simulink model "DLL_Demo"  (R2021a)
settings: Solver=VariableStepAuto  StartTime=0.0  StopTime=inf  RelTol=1e-3
settings Model: Creator=ccortez  LastModifiedBy=jdehg
settings SolverCC: AlgebraicLoopSolver=TrustRegion
settings DebuggingCC: SFMachineParentedDataDiag=warning

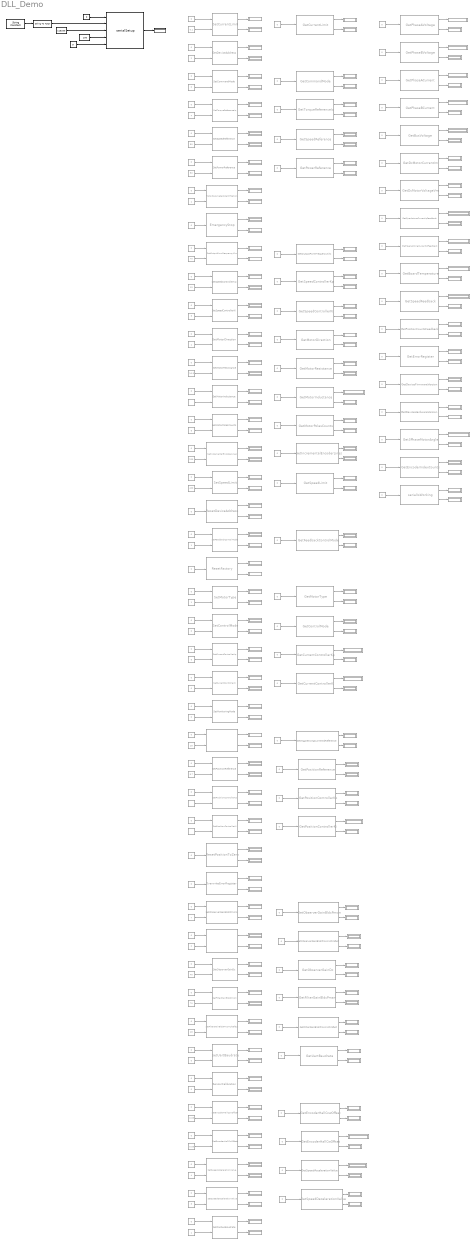
== system DLL_Demo ==
  note: Subsystem
  Constant1 : Constant  Value=115200  OutDataTypeStr=uint32
  Constant10 : Constant  Commented=on  Value=4  OutDataTypeStr=single
  Constant{2..3,6,8..9,11,15,17,19,21,23..24,26,28,30,32,34,36,38,40,42..43,45..48,50,52,54,56,58,60,62..64,66,68,70,72,74,76..78,80,82,84,86,88..136} (96 alike) : Constant  Commented=on  Value=0  OutDataTypeStr=uint8
  Constant12 : Constant  Value=100  OutDataTypeStr=double
  Constant13 : Constant  Value=5  OutDataTypeStr=int32
  Constant14 : Constant  Commented=on  Value=50  OutDataTypeStr=uint32
  Constant16 : Constant  Commented=on  Value=50  OutDataTypeStr=single
  Constant18 : Constant  Value=0  OutDataTypeStr=uint8
  Constant20 : Constant  Commented=on  OutDataTypeStr=boolean
  Constant22 : Constant  Commented=on  Value=70  OutDataTypeStr=uint32
  Constant25 : Constant  Commented=on  Value=13  OutDataTypeStr=single
  Constant27 : Constant  Commented=on  Value=9  OutDataTypeStr=single
  Constant29 : Constant  Commented=on  OutDataTypeStr=boolean
  Constant31 : Constant  Commented=on  Value=10.5  OutDataTypeStr=single
  Constant33 : Constant  Commented=on  Value=0.004  OutDataTypeStr=single
  Constant35 : Constant  Commented=on  Value=6  OutDataTypeStr=uint32
  Constant37 : Constant  Commented=on  Value=200  OutDataTypeStr=uint32
  Constant39 : Constant  Commented=on  Value=400  OutDataTypeStr=uint32
  Constant4 : Constant  Commented=on  Value=0.1  OutDataTypeStr=single
  Constant41 : Constant  Commented=on  OutDataTypeStr=uint8
  Constant44 : Constant  Commented=on  OutDataTypeStr=uint8
  Constant49 : Constant  Commented=on  Value=6  OutDataTypeStr=single
  Constant5 : Constant  Commented=on  Value=2  OutDataTypeStr=uint8
  Constant51 : Constant  Commented=on  Value=0  OutDataTypeStr=single
  Constant53 : Constant  Commented=on  Value=0  OutDataTypeStr=boolean
  Constant55 : Constant  Commented=on  Value=18  OutDataTypeStr=single
  Constant57 : Constant  Commented=on  Value=5.7  OutDataTypeStr=uint32
  Constant59 : Constant  Commented=on  Value=16.78  OutDataTypeStr=single
  Constant61 : Constant  Commented=on  Value=10.76  OutDataTypeStr=single
  Constant65 : Constant  Commented=on  Value=7  OutDataTypeStr=single
  Constant67 : Constant  Commented=on  Value=2  OutDataTypeStr=single
  Constant69 : Constant  Commented=on  Value=40  OutDataTypeStr=single
  Constant7 : Constant  Commented=on  Value=0  OutDataTypeStr=boolean
  Constant71 : Constant  Commented=on  Value=70  OutDataTypeStr=single
  Constant73 : Constant  Commented=on  Value=18  OutDataTypeStr=single
  Constant75 : Constant  Commented=on  Value=0  OutDataTypeStr=boolean
  Constant79 : Constant  Commented=on  Value=0.05  OutDataTypeStr=single
  Constant81 : Constant  Commented=on  Value=0.05  OutDataTypeStr=single
  Constant83 : Constant  Commented=on  Value=4  OutDataTypeStr=single
  Constant85 : Constant  Commented=on  Value=3  OutDataTypeStr=single
  Constant87 : Constant  Commented=on  OutDataTypeStr=uint8
  Display{1..4,6..189} (188 alike) : Display  Commented=on
      settings: Format=decimal (Stored Integer)
  Display5 : Display
      settings: Format=decimal (Stored Integer)
  S-Function Builder : S-Function  Priority=2  Commented=on  FunctionName=SetCurrentLimit  SFunctionModules=SetCurrentLimit_wrapper  SFunctionDeploymentMode=off  EnableBusSupport=off  mask(S-Function Builder){}
      mask help: Simulink:masks:SFunctionBuilder_MD
      mask init:
      | val = [[.9  0.75 0.75 1 1 .9 .9 1]',[1 1 0.75 0.75 .9 .9 1 .9]'];try , sys = get_param(gcb,'SfunBuilderFcnName');if isempty(sys), sys = get_param(gcb,'FunctionName'); end,catch, sys = get_param(gcb,'FunctionName'); end
      settings: CopyFcn=set_param(gcbh,'LinkStatus','none')  OpenFcn=sfunctionwizard(gcbh)
      mask Display: plot(val(:,1),val(:,2)),disp(sys),port_label('input',1,'Address'),port_label('input',2,'Value'),port_label('output',1,'Result'),port_label('output',2,'Error')
  S-Function Builder1 : S-Function  Priority=2  Commented=on  FunctionName=SetDeviceAddress  SFunctionModules=SetDeviceAddress_wrapper  SFunctionDeploymentMode=off  EnableBusSupport=off  mask(S-Function Builder){}
      mask help: Simulink:masks:SFunctionBuilder_MD
      mask init: same as DLL_Demo/S-Function Builder
      settings: CopyFcn=set_param(gcbh,'LinkStatus','none')  OpenFcn=sfunctionwizard(gcbh)
      mask Display: plot(val(:,1),val(:,2)),disp(sys),port_label('input',1,'Address'),port_label('input',2,'Value'),port_label('output',1,'Result'),port_label('output',2,'Error')
  S-Function Builder10 : S-Function  Priority=2  Commented=on  FunctionName=MotorParametersIdentification  SFunctionModules=MotorParametersIdentification_wrapper  SFunctionDeploymentMode=off  EnableBusSupport=off  mask(S-Function Builder){}
      mask help: Simulink:masks:SFunctionBuilder_MD
      mask init: same as DLL_Demo/S-Function Builder
      settings: CopyFcn=set_param(gcbh,'LinkStatus','none')  OpenFcn=sfunctionwizard(gcbh)
      mask Display: plot(val(:,1),val(:,2)),disp(sys),port_label('input',1,'Address'),port_label('input',2,'Value'),port_label('output',1,'Result'),port_label('output',2,'Error')
  S-Function Builder11 : S-Function  Priority=2  Commented=on  FunctionName=EmergencyStop  SFunctionModules=EmergencyStop_wrapper  SFunctionDeploymentMode=off  EnableBusSupport=off  mask(S-Function Builder){}
      mask help: Simulink:masks:SFunctionBuilder_MD
      mask init: same as DLL_Demo/S-Function Builder
      settings: CopyFcn=set_param(gcbh,'LinkStatus','none')  OpenFcn=sfunctionwizard(gcbh)
      mask Display:
      | plot(val(:,1),val(:,2))
      | disp(sys)
      | port_label('input',1,'Address')
      | port_label('output',1,'Result')
      | port_label('output',2,'Error')
  S-Function Builder12 : S-Function  Priority=2  Commented=on  FunctionName=SetOutputPwmFrequencyKhz  SFunctionModules=SetOutputPwmFrequencyKhz_wrapper  SFunctionDeploymentMode=off  EnableBusSupport=off  mask(S-Function Builder){}
      mask help: Simulink:masks:SFunctionBuilder_MD
      mask init: same as DLL_Demo/S-Function Builder
      settings: CopyFcn=set_param(gcbh,'LinkStatus','none')  OpenFcn=sfunctionwizard(gcbh)
      mask Display:
      | plot(val(:,1),val(:,2))
      | disp(sys)
      | port_label('input',1,'Address')
      | port_label('input',2,'Value')
      | port_label('output',1,'Result')
      | port_label('output',2,'Error')
  S-Function Builder13 : S-Function  Priority=2  Commented=on  FunctionName=SetSpeedControllerKp  SFunctionModules=SetSpeedControllerKp_wrapper  SFunctionDeploymentMode=off  EnableBusSupport=off  mask(S-Function Builder){}
      mask help: Simulink:masks:SFunctionBuilder_MD
      mask init: same as DLL_Demo/S-Function Builder
      settings: CopyFcn=set_param(gcbh,'LinkStatus','none')  OpenFcn=sfunctionwizard(gcbh)
      mask Display: plot(val(:,1),val(:,2)),disp(sys),port_label('input',1,'Address'),port_label('input',2,'Value'),port_label('output',1,'Result'),port_label('output',2,'Error')
  S-Function Builder14 : S-Function  Priority=2  Commented=on  FunctionName=SetSpeedControllerKi  SFunctionModules=SetSpeedControllerKi_wrapper  SFunctionDeploymentMode=off  EnableBusSupport=off  mask(S-Function Builder){}
      mask help: Simulink:masks:SFunctionBuilder_MD
      mask init: same as DLL_Demo/S-Function Builder
      settings: CopyFcn=set_param(gcbh,'LinkStatus','none')  OpenFcn=sfunctionwizard(gcbh)
      mask Display: plot(val(:,1),val(:,2)),disp(sys),port_label('input',1,'Address'),port_label('input',2,'Value'),port_label('output',1,'Result'),port_label('output',2,'Error')
  S-Function Builder15 : S-Function  Priority=2  Commented=on  FunctionName=SetMotorDirection  SFunctionModules=SetMotorDirection_wrapper  SFunctionDeploymentMode=off  EnableBusSupport=off  mask(S-Function Builder){}
      mask help: Simulink:masks:SFunctionBuilder_MD
      mask init: same as DLL_Demo/S-Function Builder
      settings: CopyFcn=set_param(gcbh,'LinkStatus','none')  OpenFcn=sfunctionwizard(gcbh)
      mask Display: plot(val(:,1),val(:,2)),disp(sys),port_label('input',1,'Address'),port_label('input',2,'Value'),port_label('output',1,'Result'),port_label('output',2,'Error')
  S-Function Builder16 : S-Function  Priority=2  Commented=on  FunctionName=SetMotorResistance  SFunctionModules=SetMotorResistance_wrapper  SFunctionDeploymentMode=off  EnableBusSupport=off  mask(S-Function Builder){}
      mask help: Simulink:masks:SFunctionBuilder_MD
      mask init: same as DLL_Demo/S-Function Builder
      settings: CopyFcn=set_param(gcbh,'LinkStatus','none')  OpenFcn=sfunctionwizard(gcbh)
      mask Display: plot(val(:,1),val(:,2)),disp(sys),port_label('input',1,'Address'),port_label('input',2,'Value'),port_label('output',1,'Result'),port_label('output',2,'Error')
  S-Function Builder17 : S-Function  Priority=2  Commented=on  FunctionName=SetMotorInductance  SFunctionModules=SetMotorInductance_wrapper  SFunctionDeploymentMode=off  EnableBusSupport=off  mask(S-Function Builder){}
      mask help: Simulink:masks:SFunctionBuilder_MD
      mask init: same as DLL_Demo/S-Function Builder
      settings: CopyFcn=set_param(gcbh,'LinkStatus','none')  OpenFcn=sfunctionwizard(gcbh)
      mask Display: plot(val(:,1),val(:,2)),disp(sys),port_label('input',1,'Address'),port_label('input',2,'Value'),port_label('output',1,'Result'),port_label('output',2,'Error')
  S-Function Builder18 : S-Function  Priority=2  Commented=on  FunctionName=SetMotorPolesCounts  SFunctionModules=SetMotorPolesCounts_wrapper  SFunctionDeploymentMode=off  EnableBusSupport=off  mask(S-Function Builder){}
      mask help: Simulink:masks:SFunctionBuilder_MD
      mask init: same as DLL_Demo/S-Function Builder
      settings: CopyFcn=set_param(gcbh,'LinkStatus','none')  OpenFcn=sfunctionwizard(gcbh)
      mask Display:
      | plot(val(:,1),val(:,2))
      | disp(sys)
      | port_label('input',1,'Address')
      | port_label('input',2,'Value')
      | port_label('output',1,'Result')
      | port_label('output',2,'Error')
  S-Function Builder19 : S-Function  Priority=2  Commented=on  FunctionName=SetIncrementalEncoderLines  SFunctionModules=SetIncrementalEncoderLines_wrapper  SFunctionDeploymentMode=off  EnableBusSupport=off  mask(S-Function Builder){}
      mask help: Simulink:masks:SFunctionBuilder_MD
      mask init: same as DLL_Demo/S-Function Builder
      settings: CopyFcn=set_param(gcbh,'LinkStatus','none')  OpenFcn=sfunctionwizard(gcbh)
      mask Display:
      | plot(val(:,1),val(:,2))
      | disp(sys)
      | port_label('input',1,'Address')
      | port_label('input',2,'Value')
      | port_label('output',1,'Result')
      | port_label('output',2,'Error')
  S-Function Builder2 : S-Function  Priority=2  Commented=on  FunctionName=SetCommandMode  SFunctionModules=SetCommandMode_wrapper  SFunctionDeploymentMode=off  EnableBusSupport=off  mask(S-Function Builder){}
      mask help: Simulink:masks:SFunctionBuilder_MD
      mask init: same as DLL_Demo/S-Function Builder
      settings: CopyFcn=set_param(gcbh,'LinkStatus','none')  OpenFcn=sfunctionwizard(gcbh)
      mask Display: plot(val(:,1),val(:,2)),disp(sys),port_label('input',1,'Address'),port_label('input',2,'Value'),port_label('output',1,'Result'),port_label('output',2,'Error')
  S-Function Builder20 : S-Function  Priority=2  Commented=on  FunctionName=SetSpeedLimit  SFunctionModules=SetSpeedLimit_wrapper  SFunctionDeploymentMode=off  EnableBusSupport=off  mask(S-Function Builder){}
      mask help: Simulink:masks:SFunctionBuilder_MD
      mask init: same as DLL_Demo/S-Function Builder
      settings: CopyFcn=set_param(gcbh,'LinkStatus','none')  OpenFcn=sfunctionwizard(gcbh)
      mask Display:
      | plot(val(:,1),val(:,2))
      | disp(sys)
      | port_label('input',1,'Address')
      | port_label('input',2,'Value')
      | port_label('output',1,'Result')
      | port_label('output',2,'Error')
  S-Function Builder21 : S-Function  Priority=2  Commented=on  FunctionName=SetFeedbackControlMode  SFunctionModules=SetFeedbackControlMode_wrapper  SFunctionDeploymentMode=off  EnableBusSupport=off  mask(S-Function Builder){}
      mask help: Simulink:masks:SFunctionBuilder_MD
      mask init: same as DLL_Demo/S-Function Builder
      settings: CopyFcn=set_param(gcbh,'LinkStatus','none')  OpenFcn=sfunctionwizard(gcbh)
      mask Display: plot(val(:,1),val(:,2)),disp(sys),port_label('input',1,'Address'),port_label('input',2,'Value'),port_label('output',1,'Result'),port_label('output',2,'Error')
  S-Function Builder22 : S-Function  Priority=2  Commented=on  FunctionName=ResetDeviceAddress  SFunctionModules=ResetDeviceAddress_wrapper  SFunctionDeploymentMode=off  EnableBusSupport=off  mask(S-Function Builder){}
      mask help: Simulink:masks:SFunctionBuilder_MD
      mask init: same as DLL_Demo/S-Function Builder
      settings: CopyFcn=set_param(gcbh,'LinkStatus','none')  OpenFcn=sfunctionwizard(gcbh)
      mask Display:
      | plot(val(:,1),val(:,2))
      | disp(sys)
      | port_label('input',1,'Address')
      | port_label('output',1,'Result')
      | port_label('output',2,'Error')
  S-Function Builder23 : S-Function  Priority=2  Commented=on  FunctionName=SetMotorType  SFunctionModules=SetMotorType_wrapper  SFunctionDeploymentMode=off  EnableBusSupport=off  mask(S-Function Builder){}
      mask help: Simulink:masks:SFunctionBuilder_MD
      mask init: same as DLL_Demo/S-Function Builder
      settings: CopyFcn=set_param(gcbh,'LinkStatus','none')  OpenFcn=sfunctionwizard(gcbh)
      mask Display: plot(val(:,1),val(:,2)),disp(sys),port_label('input',1,'Address'),port_label('input',2,'Value'),port_label('output',1,'Result'),port_label('output',2,'Error')
  S-Function Builder24 : S-Function  Priority=2  Commented=on  FunctionName=ResetFactory  SFunctionModules=ResetFactory_wrapper  SFunctionDeploymentMode=off  EnableBusSupport=off  mask(S-Function Builder){}
      mask help: Simulink:masks:SFunctionBuilder_MD
      mask init: same as DLL_Demo/S-Function Builder
      settings: CopyFcn=set_param(gcbh,'LinkStatus','none')  OpenFcn=sfunctionwizard(gcbh)
      mask Display:
      | plot(val(:,1),val(:,2))
      | disp(sys)
      | port_label('input',1,'Address')
      | port_label('output',1,'Result')
      | port_label('output',2,'Error')
  S-Function Builder25 : S-Function  Priority=2  Commented=on  FunctionName=SetControlMode  SFunctionModules=SetControlMode_wrapper  SFunctionDeploymentMode=off  EnableBusSupport=off  mask(S-Function Builder){}
      mask help: Simulink:masks:SFunctionBuilder_MD
      mask init: same as DLL_Demo/S-Function Builder
      settings: CopyFcn=set_param(gcbh,'LinkStatus','none')  OpenFcn=sfunctionwizard(gcbh)
      mask Display: plot(val(:,1),val(:,2)),disp(sys),port_label('input',1,'Address'),port_label('input',2,'Value'),port_label('output',1,'Result'),port_label('output',2,'Error')
  S-Function Builder26 : S-Function  Priority=2  Commented=on  FunctionName=SetCurrentControllerKp  SFunctionModules=SetCurrentControllerKp_wrapper  SFunctionDeploymentMode=off  EnableBusSupport=off  mask(S-Function Builder){}
      mask help: Simulink:masks:SFunctionBuilder_MD
      mask init: same as DLL_Demo/S-Function Builder
      settings: CopyFcn=set_param(gcbh,'LinkStatus','none')  OpenFcn=sfunctionwizard(gcbh)
      mask Display: plot(val(:,1),val(:,2)),disp(sys),port_label('input',1,'Address'),port_label('input',2,'Value'),port_label('output',1,'Result'),port_label('output',2,'Error')
  S-Function Builder27 : S-Function  Priority=2  Commented=on  FunctionName=SetCurrentControllerKi  SFunctionModules=SetCurrentControllerKi_wrapper  SFunctionDeploymentMode=off  EnableBusSupport=off  mask(S-Function Builder){}
      mask help: Simulink:masks:SFunctionBuilder_MD
      mask init: same as DLL_Demo/S-Function Builder
      settings: CopyFcn=set_param(gcbh,'LinkStatus','none')  OpenFcn=sfunctionwizard(gcbh)
      mask Display: plot(val(:,1),val(:,2)),disp(sys),port_label('input',1,'Address'),port_label('input',2,'Value'),port_label('output',1,'Result'),port_label('output',2,'Error')
  S-Function Builder28 : S-Function  Priority=2  Commented=on  FunctionName=SetMonitoringMode  SFunctionModules=SetMonitoringMode_wrapper  SFunctionDeploymentMode=off  EnableBusSupport=off  mask(S-Function Builder){}
      mask help: Simulink:masks:SFunctionBuilder_MD
      mask init: same as DLL_Demo/S-Function Builder
      settings: CopyFcn=set_param(gcbh,'LinkStatus','none')  OpenFcn=sfunctionwizard(gcbh)
      mask Display: plot(val(:,1),val(:,2)),disp(sys),port_label('input',1,'Address'),port_label('input',2,'Value'),port_label('output',1,'Result'),port_label('output',2,'Error')
  S-Function Builder29 : S-Function  Priority=2  Commented=on  FunctionName=SetMagnetizingCurrentIdReference  SFunctionModules=SetMagnetizingCurrentIdReference_wrapper  SFunctionDeploymentMode=off  EnableBusSupport=off  mask(S-Function Builder){}
      mask help: Simulink:masks:SFunctionBuilder_MD
      mask init: same as DLL_Demo/S-Function Builder
      settings: CopyFcn=set_param(gcbh,'LinkStatus','none')  OpenFcn=sfunctionwizard(gcbh)
      mask Display: plot(val(:,1),val(:,2)),disp(sys),port_label('input',1,'Address'),port_label('input',2,'Value'),port_label('output',1,'Result'),port_label('output',2,'Error')
  S-Function Builder3 : S-Function  Priority=3  Commented=on  FunctionName=GetCommandMode  SFunctionModules=GetCommandMode_wrapper  SFunctionDeploymentMode=off  EnableBusSupport=off  mask(S-Function Builder){}
      mask help: Simulink:masks:SFunctionBuilder_MD
      mask init: same as DLL_Demo/S-Function Builder
      settings: CopyFcn=set_param(gcbh,'LinkStatus','none')  OpenFcn=sfunctionwizard(gcbh)
      mask Display: plot(val(:,1),val(:,2)),disp(sys),port_label('input',1,'Address'),port_label('output',1,'Result'),port_label('output',2,'Error')
  S-Function Builder30 : S-Function  Priority=2  Commented=on  FunctionName=SetPositionReference  SFunctionModules=SetPositionReference_wrapper  SFunctionDeploymentMode=off  EnableBusSupport=off  mask(S-Function Builder){}
      mask help: Simulink:masks:SFunctionBuilder_MD
      mask init: same as DLL_Demo/S-Function Builder
      settings: CopyFcn=set_param(gcbh,'LinkStatus','none')  OpenFcn=sfunctionwizard(gcbh)
      mask Display:
      | plot(val(:,1),val(:,2))
      | disp(sys)
      | port_label('input',1,'Address')
      | port_label('input',2,'Value')
      | port_label('output',1,'Result')
      | port_label('output',2,'Error')
  S-Function Builder31 : S-Function  Priority=2  Commented=on  FunctionName=SetPositionControllerKp  SFunctionModules=SetPositionControllerKp_wrapper  SFunctionDeploymentMode=off  EnableBusSupport=off  mask(S-Function Builder){}
      mask help: Simulink:masks:SFunctionBuilder_MD
      mask init: same as DLL_Demo/S-Function Builder
      settings: CopyFcn=set_param(gcbh,'LinkStatus','none')  OpenFcn=sfunctionwizard(gcbh)
      mask Display: plot(val(:,1),val(:,2)),disp(sys),port_label('input',1,'Address'),port_label('input',2,'Value'),port_label('output',1,'Result'),port_label('output',2,'Error')
  S-Function Builder32 : S-Function  Priority=2  Commented=on  FunctionName=SetPositionControllerKi  SFunctionModules=SetPositionControllerKi_wrapper  SFunctionDeploymentMode=off  EnableBusSupport=off  mask(S-Function Builder){}
      mask help: Simulink:masks:SFunctionBuilder_MD
      mask init: same as DLL_Demo/S-Function Builder
      settings: CopyFcn=set_param(gcbh,'LinkStatus','none')  OpenFcn=sfunctionwizard(gcbh)
      mask Display: plot(val(:,1),val(:,2)),disp(sys),port_label('input',1,'Address'),port_label('input',2,'Value'),port_label('output',1,'Result'),port_label('output',2,'Error')
  S-Function Builder33 : S-Function  Priority=2  Commented=on  FunctionName=ResetPositionToZero  SFunctionModules=ResetPositionToZero_wrapper  SFunctionDeploymentMode=off  EnableBusSupport=off  mask(S-Function Builder){}
      mask help: Simulink:masks:SFunctionBuilder_MD
      mask init: same as DLL_Demo/S-Function Builder
      settings: CopyFcn=set_param(gcbh,'LinkStatus','none')  OpenFcn=sfunctionwizard(gcbh)
      mask Display:
      | plot(val(:,1),val(:,2))
      | disp(sys)
      | port_label('input',1,'Address')
      | port_label('output',1,'Result')
      | port_label('output',2,'Error')
  S-Function Builder34 : S-Function  Priority=2  Commented=on  FunctionName=OverwriteErrorRegister  SFunctionModules=OverwriteErrorRegister_wrapper  SFunctionDeploymentMode=off  EnableBusSupport=off  mask(S-Function Builder){}
      mask help: Simulink:masks:SFunctionBuilder_MD
      mask init: same as DLL_Demo/S-Function Builder
      settings: CopyFcn=set_param(gcbh,'LinkStatus','none')  OpenFcn=sfunctionwizard(gcbh)
      mask Display:
      | plot(val(:,1),val(:,2))
      | disp(sys)
      | port_label('input',1,'Address')
      | port_label('output',1,'Result')
      | port_label('output',2,'Error')
  S-Function Builder35 : S-Function  Priority=2  Commented=on  FunctionName=SetObserverGainBldcPmsm  SFunctionModules=SetObserverGainBldcPmsm_wrapper  SFunctionDeploymentMode=off  EnableBusSupport=off  mask(S-Function Builder){}
      mask help: Simulink:masks:SFunctionBuilder_MD
      mask init: same as DLL_Demo/S-Function Builder
      settings: CopyFcn=set_param(gcbh,'LinkStatus','none')  OpenFcn=sfunctionwizard(gcbh)
      mask Display: plot(val(:,1),val(:,2)),disp(sys),port_label('input',1,'Address'),port_label('input',2,'Value'),port_label('output',1,'Result'),port_label('output',2,'Error')
  S-Function Builder36 : S-Function  Priority=2  Commented=on  FunctionName=SetObserverGainBldcPmsmUltrafast  SFunctionModules=SetObserverGainBldcPmsmUltrafast_wrapper  SFunctionDeploymentMode=off  EnableBusSupport=off  mask(S-Function Builder){}
      mask help: Simulink:masks:SFunctionBuilder_MD
      mask init: same as DLL_Demo/S-Function Builder
      settings: CopyFcn=set_param(gcbh,'LinkStatus','none')  OpenFcn=sfunctionwizard(gcbh)
      mask Display: plot(val(:,1),val(:,2)),disp(sys),port_label('input',1,'Address'),port_label('input',2,'Value'),port_label('output',1,'Result'),port_label('output',2,'Error')
  S-Function Builder37 : S-Function  Priority=2  Commented=on  FunctionName=SetObserverGainDc  SFunctionModules=SetObserverGainDc_wrapper  SFunctionDeploymentMode=off  EnableBusSupport=off  mask(S-Function Builder){}
      mask help: Simulink:masks:SFunctionBuilder_MD
      mask init: same as DLL_Demo/S-Function Builder
      settings: CopyFcn=set_param(gcbh,'LinkStatus','none')  OpenFcn=sfunctionwizard(gcbh)
      mask Display: plot(val(:,1),val(:,2)),disp(sys),port_label('input',1,'Address'),port_label('input',2,'Value'),port_label('output',1,'Result'),port_label('output',2,'Error')
  S-Function Builder38 : S-Function  Priority=2  Commented=on  FunctionName=SetFilterGainBldcPmsm  SFunctionModules=SetFilterGainBldcPmsm_wrapper  SFunctionDeploymentMode=off  EnableBusSupport=off  mask(S-Function Builder){}
      mask help: Simulink:masks:SFunctionBuilder_MD
      mask init: same as DLL_Demo/S-Function Builder
      settings: CopyFcn=set_param(gcbh,'LinkStatus','none')  OpenFcn=sfunctionwizard(gcbh)
      mask Display: plot(val(:,1),val(:,2)),disp(sys),port_label('input',1,'Address'),port_label('input',2,'Value'),port_label('output',1,'Result'),port_label('output',2,'Error')
  S-Function Builder39 : S-Function  Priority=2  Commented=on  FunctionName=SetFilterGainBldcPmsmUltrafast  SFunctionModules=SetFilterGainBldcPmsmUltrafast_wrapper  SFunctionDeploymentMode=off  EnableBusSupport=off  mask(S-Function Builder){}
      mask help: Simulink:masks:SFunctionBuilder_MD
      mask init: same as DLL_Demo/S-Function Builder
      settings: CopyFcn=set_param(gcbh,'LinkStatus','none')  OpenFcn=sfunctionwizard(gcbh)
      mask Display: plot(val(:,1),val(:,2)),disp(sys),port_label('input',1,'Address'),port_label('input',2,'Value'),port_label('output',1,'Result'),port_label('output',2,'Error')
  S-Function Builder4 : S-Function  Priority=2  Commented=on  FunctionName=SetTorqueReferenceIq  SFunctionModules=SetTorqueReferenceIq_wrapper  SFunctionDeploymentMode=off  EnableBusSupport=off  mask(S-Function Builder){}
      mask help: Simulink:masks:SFunctionBuilder_MD
      mask init: same as DLL_Demo/S-Function Builder
      settings: CopyFcn=set_param(gcbh,'LinkStatus','none')  OpenFcn=sfunctionwizard(gcbh)
      mask Display: plot(val(:,1),val(:,2)),disp(sys),port_label('input',1,'Address'),port_label('input',2,'Value'),port_label('output',1,'Result'),port_label('output',2,'Error')
  S-Function Builder40 : S-Function  Priority=2  Commented=on  FunctionName=SetUartBaudrate  SFunctionModules=SetUartBaudrate_wrapper  SFunctionDeploymentMode=off  EnableBusSupport=off  mask(S-Function Builder){}
      mask help: Simulink:masks:SFunctionBuilder_MD
      mask init: same as DLL_Demo/S-Function Builder
      settings: CopyFcn=set_param(gcbh,'LinkStatus','none')  OpenFcn=sfunctionwizard(gcbh)
      mask Display: plot(val(:,1),val(:,2)),disp(sys),port_label('input',1,'Address'),port_label('input',2,'Value'),port_label('output',1,'Result'),port_label('output',2,'Error')
  S-Function Builder41 : S-Function  Priority=2  Commented=on  FunctionName=SensorCalibration  SFunctionModules=SensorCalibration_wrapper  SFunctionDeploymentMode=off  EnableBusSupport=off  mask(S-Function Builder){}
      mask help: Simulink:masks:SFunctionBuilder_MD
      mask init: same as DLL_Demo/S-Function Builder
      settings: CopyFcn=set_param(gcbh,'LinkStatus','none')  OpenFcn=sfunctionwizard(gcbh)
      mask Display: plot(val(:,1),val(:,2)),disp(sys),port_label('input',1,'Address'),port_label('input',2,'Value'),port_label('output',1,'Result'),port_label('output',2,'Error')
  S-Function Builder42 : S-Function  Priority=2  Commented=on  FunctionName=SetEncoderHallCcwOffset  SFunctionModules=SetEncoderHallCcwOffset_wrapper  SFunctionDeploymentMode=off  EnableBusSupport=off  mask(S-Function Builder){}
      mask help: Simulink:masks:SFunctionBuilder_MD
      mask init: same as DLL_Demo/S-Function Builder
      settings: CopyFcn=set_param(gcbh,'LinkStatus','none')  OpenFcn=sfunctionwizard(gcbh)
      mask Display: plot(val(:,1),val(:,2)),disp(sys),port_label('input',1,'Address'),port_label('input',2,'Value'),port_label('output',1,'Result'),port_label('output',2,'Error')
  S-Function Builder43 : S-Function  Priority=2  Commented=on  FunctionName=SetEncoderHallCwOffset  SFunctionModules=SetEncoderHallCwOffset_wrapper  SFunctionDeploymentMode=off  EnableBusSupport=off  mask(S-Function Builder){}
      mask help: Simulink:masks:SFunctionBuilder_MD
      mask init: same as DLL_Demo/S-Function Builder
      settings: CopyFcn=set_param(gcbh,'LinkStatus','none')  OpenFcn=sfunctionwizard(gcbh)
      mask Display: plot(val(:,1),val(:,2)),disp(sys),port_label('input',1,'Address'),port_label('input',2,'Value'),port_label('output',1,'Result'),port_label('output',2,'Error')
  S-Function Builder44 : S-Function  Priority=2  Commented=on  FunctionName=SetSpeedAccelerationValue  SFunctionModules=SetSpeedAccelerationValue_wrapper  SFunctionDeploymentMode=off  EnableBusSupport=off  mask(S-Function Builder){}
      mask help: Simulink:masks:SFunctionBuilder_MD
      mask init: same as DLL_Demo/S-Function Builder
      settings: CopyFcn=set_param(gcbh,'LinkStatus','none')  OpenFcn=sfunctionwizard(gcbh)
      mask Display: plot(val(:,1),val(:,2)),disp(sys),port_label('input',1,'Address'),port_label('input',2,'Value'),port_label('output',1,'Result'),port_label('output',2,'Error')
  S-Function Builder45 : S-Function  Priority=2  Commented=on  FunctionName=SetSpeedDecelerationValue  SFunctionModules=SetSpeedDecelerationValue_wrapper  SFunctionDeploymentMode=off  EnableBusSupport=off  mask(S-Function Builder){}
      mask help: Simulink:masks:SFunctionBuilder_MD
      mask init: same as DLL_Demo/S-Function Builder
      settings: CopyFcn=set_param(gcbh,'LinkStatus','none')  OpenFcn=sfunctionwizard(gcbh)
      mask Display: plot(val(:,1),val(:,2)),disp(sys),port_label('input',1,'Address'),port_label('input',2,'Value'),port_label('output',1,'Result'),port_label('output',2,'Error')
  S-Function Builder46 : S-Function  Priority=2  Commented=on  FunctionName=SetCanbusBoudrate  SFunctionModules=SetCanbusBoudrate_wrapper  SFunctionDeploymentMode=off  EnableBusSupport=off  mask(S-Function Builder){}
      mask help: Simulink:masks:SFunctionBuilder_MD
      mask init: same as DLL_Demo/S-Function Builder
      settings: CopyFcn=set_param(gcbh,'LinkStatus','none')  OpenFcn=sfunctionwizard(gcbh)
      mask Display: plot(val(:,1),val(:,2)),disp(sys),port_label('input',1,'Address'),port_label('input',2,'Value'),port_label('output',1,'Result'),port_label('output',2,'Error')
  S-Function Builder47 : S-Function  Priority=3  Commented=on  FunctionName=GetPhaseAVoltage  SFunctionModules=GetPhaseAVoltage_wrapper  SFunctionDeploymentMode=off  EnableBusSupport=off  mask(S-Function Builder){}
      mask help: Simulink:masks:SFunctionBuilder_MD
      mask init: same as DLL_Demo/S-Function Builder
      settings: CopyFcn=set_param(gcbh,'LinkStatus','none')  OpenFcn=sfunctionwizard(gcbh)
      mask Display:
      | plot(val(:,1),val(:,2))
      | disp(sys)
      | port_label('input',1,'Address')
      | port_label('output',1,'Result')
      | port_label('output',2,'Error')
  S-Function Builder48 : S-Function  Priority=3  Commented=on  FunctionName=GetPhaseBVoltage  SFunctionModules=GetPhaseBVoltage_wrapper  SFunctionDeploymentMode=off  EnableBusSupport=off  mask(S-Function Builder){}
      mask help: Simulink:masks:SFunctionBuilder_MD
      mask init: same as DLL_Demo/S-Function Builder
      settings: CopyFcn=set_param(gcbh,'LinkStatus','none')  OpenFcn=sfunctionwizard(gcbh)
      mask Display:
      | plot(val(:,1),val(:,2))
      | disp(sys)
      | port_label('input',1,'Address')
      | port_label('output',1,'Result')
      | port_label('output',2,'Error')
  S-Function Builder49 : S-Function  Priority=3  Commented=on  FunctionName=GetPhaseACurrent  SFunctionModules=GetPhaseACurrent_wrapper  SFunctionDeploymentMode=off  EnableBusSupport=off  mask(S-Function Builder){}
      mask help: Simulink:masks:SFunctionBuilder_MD
      mask init: same as DLL_Demo/S-Function Builder
      settings: CopyFcn=set_param(gcbh,'LinkStatus','none')  OpenFcn=sfunctionwizard(gcbh)
      mask Display:
      | plot(val(:,1),val(:,2))
      | disp(sys)
      | port_label('input',1,'Address')
      | port_label('output',1,'Result')
      | port_label('output',2,'Error')
  S-Function Builder5 : S-Function  Priority=1  FunctionName=serialSetup  SFunctionModules=serialSetup_wrapper  SFunctionDeploymentMode=off  EnableBusSupport=off  mask(S-Function Builder){}
      mask help: Simulink:masks:SFunctionBuilder_MD
      mask init: same as DLL_Demo/S-Function Builder
      settings: CopyFcn=set_param(gcbh,'LinkStatus','none')  OpenFcn=sfunctionwizard(gcbh)
      mask Display: plot(val(:,1),val(:,2)),disp(sys),port_label('input',1,'Address'),port_label('input',2,'COM_Port'),port_label('input',3,'Baud_Rate'),port_label('input',4,'Timeout'),port_label('input',5,'Trials_on_Failure'),port_label('output',1,'Result')
  S-Function Builder50 : S-Function  Priority=3  Commented=on  FunctionName=GetPhaseBCurrent  SFunctionModules=GetPhaseBCurrent_wrapper  SFunctionDeploymentMode=off  EnableBusSupport=off  mask(S-Function Builder){}
      mask help: Simulink:masks:SFunctionBuilder_MD
      mask init: same as DLL_Demo/S-Function Builder
      settings: CopyFcn=set_param(gcbh,'LinkStatus','none')  OpenFcn=sfunctionwizard(gcbh)
      mask Display:
      | plot(val(:,1),val(:,2))
      | disp(sys)
      | port_label('input',1,'Address')
      | port_label('output',1,'Result')
      | port_label('output',2,'Error')
  S-Function Builder51 : S-Function  Priority=3  Commented=on  FunctionName=GetBusVoltage  SFunctionModules=GetBusVoltage_wrapper  SFunctionDeploymentMode=off  EnableBusSupport=off  mask(S-Function Builder){}
      mask help: Simulink:masks:SFunctionBuilder_MD
      mask init: same as DLL_Demo/S-Function Builder
      settings: CopyFcn=set_param(gcbh,'LinkStatus','none')  OpenFcn=sfunctionwizard(gcbh)
      mask Display:
      | plot(val(:,1),val(:,2))
      | disp(sys)
      | port_label('input',1,'Address')
      | port_label('output',1,'Result')
      | port_label('output',2,'Error')
  S-Function Builder52 : S-Function  Priority=3  Commented=on  FunctionName=GetDcMotorCurrentIm  SFunctionModules=GetDcMotorCurrentIm_wrapper  SFunctionDeploymentMode=off  EnableBusSupport=off  mask(S-Function Builder){}
      mask help: Simulink:masks:SFunctionBuilder_MD
      mask init: same as DLL_Demo/S-Function Builder
      settings: CopyFcn=set_param(gcbh,'LinkStatus','none')  OpenFcn=sfunctionwizard(gcbh)
      mask Display:
      | plot(val(:,1),val(:,2))
      | disp(sys)
      | port_label('input',1,'Address')
      | port_label('output',1,'Result')
      | port_label('output',2,'Error')
  S-Function Builder53 : S-Function  Priority=3  Commented=on  FunctionName=GetDcMotorVoltageVm  SFunctionModules=GetDcMotorVoltageVm_wrapper  SFunctionDeploymentMode=off  EnableBusSupport=off  mask(S-Function Builder){}
      mask help: Simulink:masks:SFunctionBuilder_MD
      mask init: same as DLL_Demo/S-Function Builder
      settings: CopyFcn=set_param(gcbh,'LinkStatus','none')  OpenFcn=sfunctionwizard(gcbh)
      mask Display:
      | plot(val(:,1),val(:,2))
      | disp(sys)
      | port_label('input',1,'Address')
      | port_label('output',1,'Result')
      | port_label('output',2,'Error')
  S-Function Builder54 : S-Function  Priority=3  Commented=on  FunctionName=GetSpeedControllerKp  SFunctionModules=GetSpeedControllerKp_wrapper  SFunctionDeploymentMode=off  EnableBusSupport=off  mask(S-Function Builder){}
      mask help: Simulink:masks:SFunctionBuilder_MD
      mask init: same as DLL_Demo/S-Function Builder
      settings: CopyFcn=set_param(gcbh,'LinkStatus','none')  OpenFcn=sfunctionwizard(gcbh)
      mask Display:
      | plot(val(:,1),val(:,2))
      | disp(sys)
      | port_label('input',1,'Address')
      | port_label('output',1,'Result')
      | port_label('output',2,'Error')
  S-Function Builder55 : S-Function  Priority=3  Commented=on  FunctionName=GetSpeedControllerKi  SFunctionModules=GetSpeedControllerKi_wrapper  SFunctionDeploymentMode=off  EnableBusSupport=off  mask(S-Function Builder){}
      mask help: Simulink:masks:SFunctionBuilder_MD
      mask init: same as DLL_Demo/S-Function Builder
      settings: CopyFcn=set_param(gcbh,'LinkStatus','none')  OpenFcn=sfunctionwizard(gcbh)
      mask Display:
      | plot(val(:,1),val(:,2))
      | disp(sys)
      | port_label('input',1,'Address')
      | port_label('output',1,'Result')
      | port_label('output',2,'Error')
  S-Function Builder56 : S-Function  Priority=3  Commented=on  FunctionName=GetOutputPwmFrequencyKhz  SFunctionModules=GetOutputPwmFrequencyKhz_wrapper  SFunctionDeploymentMode=off  EnableBusSupport=off  mask(S-Function Builder){}
      mask help: Simulink:masks:SFunctionBuilder_MD
      mask init: same as DLL_Demo/S-Function Builder
      settings: CopyFcn=set_param(gcbh,'LinkStatus','none')  OpenFcn=sfunctionwizard(gcbh)
      mask Display:
      | plot(val(:,1),val(:,2))
      | disp(sys)
      | port_label('input',1,'Address')
      | port_label('output',1,'Result')
      | port_label('output',2,'Error')
  S-Function Builder57 : S-Function  Priority=3  Commented=on  FunctionName=GetQuadratureCurrentIqFeedback  SFunctionModules=GetQuadratureCurrentIqFeedback_wrapper  SFunctionDeploymentMode=off  EnableBusSupport=off  mask(S-Function Builder){}
      mask help: Simulink:masks:SFunctionBuilder_MD
      mask init: same as DLL_Demo/S-Function Builder
      settings: CopyFcn=set_param(gcbh,'LinkStatus','none')  OpenFcn=sfunctionwizard(gcbh)
      mask Display:
      | plot(val(:,1),val(:,2))
      | disp(sys)
      | port_label('input',1,'Address')
      | port_label('output',1,'Result')
      | port_label('output',2,'Error')
  S-Function Builder58 : S-Function  Priority=3  Commented=on  FunctionName=GetMagnetizingCurrentIdFeedback  SFunctionModules=GetMagnetizingCurrentIdFeedback_wrapper  SFunctionDeploymentMode=off  EnableBusSupport=off  mask(S-Function Builder){}
      mask help: Simulink:masks:SFunctionBuilder_MD
      mask init: same as DLL_Demo/S-Function Builder
      settings: CopyFcn=set_param(gcbh,'LinkStatus','none')  OpenFcn=sfunctionwizard(gcbh)
      mask Display:
      | plot(val(:,1),val(:,2))
      | disp(sys)
      | port_label('input',1,'Address')
      | port_label('output',1,'Result')
      | port_label('output',2,'Error')
  S-Function Builder59 : S-Function  Priority=3  Commented=on  FunctionName=GetMotorPolesCounts  SFunctionModules=GetMotorPolesCounts_wrapper  SFunctionDeploymentMode=off  EnableBusSupport=off  mask(S-Function Builder){}
      mask help: Simulink:masks:SFunctionBuilder_MD
      mask init: same as DLL_Demo/S-Function Builder
      settings: CopyFcn=set_param(gcbh,'LinkStatus','none')  OpenFcn=sfunctionwizard(gcbh)
      mask Display:
      | plot(val(:,1),val(:,2))
      | disp(sys)
      | port_label('input',1,'Address')
      | port_label('output',1,'Result')
      | port_label('output',2,'Error')
  S-Function Builder6 : S-Function  Priority=3  Commented=on  FunctionName=GetCurrentLimit  SFunctionModules=GetCurrentLimit_wrapper  SFunctionDeploymentMode=off  EnableBusSupport=off  mask(S-Function Builder){}
      mask help: Simulink:masks:SFunctionBuilder_MD
      mask init: same as DLL_Demo/S-Function Builder
      settings: CopyFcn=set_param(gcbh,'LinkStatus','none')  OpenFcn=sfunctionwizard(gcbh)
      mask Display: plot(val(:,1),val(:,2)),disp(sys),port_label('input',1,'Address'),port_label('output',1,'Result'),port_label('output',2,'Error')
  S-Function Builder60 : S-Function  Priority=3  Commented=on  FunctionName=GetIncrementalEncoderLines  SFunctionModules=GetIncrementalEncoderLines_wrapper  SFunctionDeploymentMode=off  EnableBusSupport=off  mask(S-Function Builder){}
      mask help: Simulink:masks:SFunctionBuilder_MD
      mask init: same as DLL_Demo/S-Function Builder
      settings: CopyFcn=set_param(gcbh,'LinkStatus','none')  OpenFcn=sfunctionwizard(gcbh)
      mask Display:
      | plot(val(:,1),val(:,2))
      | disp(sys)
      | port_label('input',1,'Address')
      | port_label('output',1,'Result')
      | port_label('output',2,'Error')
  S-Function Builder61 : S-Function  Priority=3  Commented=on  FunctionName=GetCurrentControllerKp  SFunctionModules=GetCurrentControllerKp_wrapper  SFunctionDeploymentMode=off  EnableBusSupport=off  mask(S-Function Builder){}
      mask help: Simulink:masks:SFunctionBuilder_MD
      mask init: same as DLL_Demo/S-Function Builder
      settings: CopyFcn=set_param(gcbh,'LinkStatus','none')  OpenFcn=sfunctionwizard(gcbh)
      mask Display:
      | plot(val(:,1),val(:,2))
      | disp(sys)
      | port_label('input',1,'Address')
      | port_label('output',1,'Result')
      | port_label('output',2,'Error')
  S-Function Builder62 : S-Function  Priority=3  Commented=on  FunctionName=GetCurrentControllerKi  SFunctionModules=GetCurrentControllerKi_wrapper  SFunctionDeploymentMode=off  EnableBusSupport=off  mask(S-Function Builder){}
      mask help: Simulink:masks:SFunctionBuilder_MD
      mask init: same as DLL_Demo/S-Function Builder
      settings: CopyFcn=set_param(gcbh,'LinkStatus','none')  OpenFcn=sfunctionwizard(gcbh)
      mask Display: plot(val(:,1),val(:,2)),disp(sys),port_label('input',1,'Address'),port_label('output',1,'Result'),port_label('output',2,'Error')
  S-Function Builder63 : S-Function  Priority=3  Commented=on  FunctionName=GetBoardTemperature  SFunctionModules=GetBoardTemperature_wrapper  SFunctionDeploymentMode=off  EnableBusSupport=off  mask(S-Function Builder){}
      mask help: Simulink:masks:SFunctionBuilder_MD
      mask init: same as DLL_Demo/S-Function Builder
      settings: CopyFcn=set_param(gcbh,'LinkStatus','none')  OpenFcn=sfunctionwizard(gcbh)
      mask Display:
      | plot(val(:,1),val(:,2))
      | disp(sys)
      | port_label('input',1,'Address')
      | port_label('output',1,'Result')
      | port_label('output',2,'Error')
  S-Function Builder64 : S-Function  Priority=3  Commented=on  FunctionName=GetMotorResistance  SFunctionModules=GetMotorResistance_wrapper  SFunctionDeploymentMode=off  EnableBusSupport=off  mask(S-Function Builder){}
      mask help: Simulink:masks:SFunctionBuilder_MD
      mask init: same as DLL_Demo/S-Function Builder
      settings: CopyFcn=set_param(gcbh,'LinkStatus','none')  OpenFcn=sfunctionwizard(gcbh)
      mask Display: plot(val(:,1),val(:,2)),disp(sys),port_label('input',1,'Address'),port_label('output',1,'Result'),port_label('output',2,'Error')
  S-Function Builder65 : S-Function  Priority=3  Commented=on  FunctionName=GetMotorInductance  SFunctionModules=GetMotorInductance_wrapper  SFunctionDeploymentMode=off  EnableBusSupport=off  mask(S-Function Builder){}
      mask help: Simulink:masks:SFunctionBuilder_MD
      mask init: same as DLL_Demo/S-Function Builder
      settings: CopyFcn=set_param(gcbh,'LinkStatus','none')  OpenFcn=sfunctionwizard(gcbh)
      mask Display: plot(val(:,1),val(:,2)),disp(sys),port_label('input',1,'Address'),port_label('output',1,'Result'),port_label('output',2,'Error')
  S-Function Builder66 : S-Function  Priority=3  Commented=on  FunctionName=GetSpeedFeedback  SFunctionModules=GetSpeedFeedback_wrapper  SFunctionDeploymentMode=off  EnableBusSupport=off  mask(S-Function Builder){}
      mask help: Simulink:masks:SFunctionBuilder_MD
      mask init: same as DLL_Demo/S-Function Builder
      settings: CopyFcn=set_param(gcbh,'LinkStatus','none')  OpenFcn=sfunctionwizard(gcbh)
      mask Display: plot(val(:,1),val(:,2)),disp(sys),port_label('input',1,'Address'),port_label('output',1,'Result'),port_label('output',2,'Error')
  S-Function Builder67 : S-Function  Priority=3  Commented=on  FunctionName=GetMotorType  SFunctionModules=GetMotorType_wrapper  SFunctionDeploymentMode=off  EnableBusSupport=off  mask(S-Function Builder){}
      mask help: Simulink:masks:SFunctionBuilder_MD
      mask init: same as DLL_Demo/S-Function Builder
      settings: CopyFcn=set_param(gcbh,'LinkStatus','none')  OpenFcn=sfunctionwizard(gcbh)
      mask Display: plot(val(:,1),val(:,2)),disp(sys),port_label('input',1,'Address'),port_label('output',1,'Result'),port_label('output',2,'Error')
  S-Function Builder68 : S-Function  Priority=3  Commented=on  FunctionName=GetFeedbackControlMode  SFunctionModules=GetFeedbackControlMode_wrapper  SFunctionDeploymentMode=off  EnableBusSupport=off  mask(S-Function Builder){}
      mask help: Simulink:masks:SFunctionBuilder_MD
      mask init: same as DLL_Demo/S-Function Builder
      settings: CopyFcn=set_param(gcbh,'LinkStatus','none')  OpenFcn=sfunctionwizard(gcbh)
      mask Display: plot(val(:,1),val(:,2)),disp(sys),port_label('input',1,'Address'),port_label('output',1,'Result'),port_label('output',2,'Error')
  S-Function Builder69 : S-Function  Priority=3  Commented=on  FunctionName=GetControlMode  SFunctionModules=GetControlMode_wrapper  SFunctionDeploymentMode=off  EnableBusSupport=off  mask(S-Function Builder){}
      mask help: Simulink:masks:SFunctionBuilder_MD
      mask init: same as DLL_Demo/S-Function Builder
      settings: CopyFcn=set_param(gcbh,'LinkStatus','none')  OpenFcn=sfunctionwizard(gcbh)
      mask Display: plot(val(:,1),val(:,2)),disp(sys),port_label('input',1,'Address'),port_label('output',1,'Result'),port_label('output',2,'Error')
  S-Function Builder7 : S-Function  Priority=3  Commented=on  FunctionName=GetTorqueReferenceIq  SFunctionModules=GetTorqueReferenceIq_wrapper  SFunctionDeploymentMode=off  EnableBusSupport=off  mask(S-Function Builder){}
      mask help: Simulink:masks:SFunctionBuilder_MD
      mask init: same as DLL_Demo/S-Function Builder
      settings: CopyFcn=set_param(gcbh,'LinkStatus','none')  OpenFcn=sfunctionwizard(gcbh)
      mask Display: plot(val(:,1),val(:,2)),disp(sys),port_label('input',1,'Address'),port_label('output',1,'Result'),port_label('output',2,'Error')
  S-Function Builder70 : S-Function  Priority=3  Commented=on  FunctionName=GetSpeedLimit  SFunctionModules=GetSpeedLimit_wrapper  SFunctionDeploymentMode=off  EnableBusSupport=off  mask(S-Function Builder){}
      mask help: Simulink:masks:SFunctionBuilder_MD
      mask init: same as DLL_Demo/S-Function Builder
      settings: CopyFcn=set_param(gcbh,'LinkStatus','none')  OpenFcn=sfunctionwizard(gcbh)
      mask Display: plot(val(:,1),val(:,2)),disp(sys),port_label('input',1,'Address'),port_label('output',1,'Result'),port_label('output',2,'Error')
  S-Function Builder71 : S-Function  Priority=3  Commented=on  FunctionName=GetPositionControllerKp  SFunctionModules=GetPositionControllerKp_wrapper  SFunctionDeploymentMode=off  EnableBusSupport=off  mask(S-Function Builder){}
      mask help: Simulink:masks:SFunctionBuilder_MD
      mask init: same as DLL_Demo/S-Function Builder
      settings: CopyFcn=set_param(gcbh,'LinkStatus','none')  OpenFcn=sfunctionwizard(gcbh)
      mask Display:
      | plot(val(:,1),val(:,2))
      | disp(sys)
      | port_label('input',1,'Address')
      | port_label('output',1,'Result')
      | port_label('output',2,'Error')
  S-Function Builder72 : S-Function  Priority=3  Commented=on  FunctionName=GetPositionControllerKi  SFunctionModules=GetPositionControllerKi_wrapper  SFunctionDeploymentMode=off  EnableBusSupport=off  mask(S-Function Builder){}
      mask help: Simulink:masks:SFunctionBuilder_MD
      mask init: same as DLL_Demo/S-Function Builder
      settings: CopyFcn=set_param(gcbh,'LinkStatus','none')  OpenFcn=sfunctionwizard(gcbh)
      mask Display:
      | plot(val(:,1),val(:,2))
      | disp(sys)
      | port_label('input',1,'Address')
      | port_label('output',1,'Result')
      | port_label('output',2,'Error')
  S-Function Builder73 : S-Function  Priority=3  Commented=on  FunctionName=GetPositionCountsFeedback  SFunctionModules=GetPositionCountsFeedback_wrapper  SFunctionDeploymentMode=off  EnableBusSupport=off  mask(S-Function Builder){}
      mask help: Simulink:masks:SFunctionBuilder_MD
      mask init: same as DLL_Demo/S-Function Builder
      settings: CopyFcn=set_param(gcbh,'LinkStatus','none')  OpenFcn=sfunctionwizard(gcbh)
      mask Display:
      | plot(val(:,1),val(:,2))
      | disp(sys)
      | port_label('input',1,'Address')
      | port_label('output',1,'Result')
      | port_label('output',2,'Error')
  S-Function Builder74 : S-Function  Priority=3  Commented=on  FunctionName=GetErrorRegister  SFunctionModules=GetErrorRegister_wrapper  SFunctionDeploymentMode=off  EnableBusSupport=off  mask(S-Function Builder){}
      mask help: Simulink:masks:SFunctionBuilder_MD
      mask init: same as DLL_Demo/S-Function Builder
      settings: CopyFcn=set_param(gcbh,'LinkStatus','none')  OpenFcn=sfunctionwizard(gcbh)
      mask Display:
      | plot(val(:,1),val(:,2))
      | disp(sys)
      | port_label('input',1,'Address')
      | port_label('output',1,'Result')
      | port_label('output',2,'Error')
  S-Function Builder75 : S-Function  Priority=3  Commented=on  FunctionName=GetDeviceFirmwareVersion  SFunctionModules=GetDeviceFirmwareVersion_wrapper  SFunctionDeploymentMode=off  EnableBusSupport=off  mask(S-Function Builder){}
      mask help: Simulink:masks:SFunctionBuilder_MD
      mask init: same as DLL_Demo/S-Function Builder
      settings: CopyFcn=set_param(gcbh,'LinkStatus','none')  OpenFcn=sfunctionwizard(gcbh)
      mask Display:
      | plot(val(:,1),val(:,2))
      | disp(sys)
      | port_label('input',1,'Address')
      | port_label('output',1,'Result')
      | port_label('output',2,'Error')
  S-Function Builder76 : S-Function  Priority=3  Commented=on  FunctionName=GetDeviceHardwareVersion  SFunctionModules=GetDeviceHardwareVersion_wrapper  SFunctionDeploymentMode=off  EnableBusSupport=off  mask(S-Function Builder){}
      mask help: Simulink:masks:SFunctionBuilder_MD
      mask init: same as DLL_Demo/S-Function Builder
      settings: CopyFcn=set_param(gcbh,'LinkStatus','none')  OpenFcn=sfunctionwizard(gcbh)
      mask Display:
      | plot(val(:,1),val(:,2))
      | disp(sys)
      | port_label('input',1,'Address')
      | port_label('output',1,'Result')
      | port_label('output',2,'Error')
  S-Function Builder77 : S-Function  Priority=3  Commented=on  FunctionName=GetMagnetizingCurrentIdReference  SFunctionModules=GetMagnetizingCurrentIdReference_wrapper  SFunctionDeploymentMode=off  EnableBusSupport=off  mask(S-Function Builder){}
      mask help: Simulink:masks:SFunctionBuilder_MD
      mask init: same as DLL_Demo/S-Function Builder
      settings: CopyFcn=set_param(gcbh,'LinkStatus','none')  OpenFcn=sfunctionwizard(gcbh)
      mask Display: plot(val(:,1),val(:,2)),disp(sys),port_label('input',1,'Address'),port_label('output',1,'Result'),port_label('output',2,'Error')
  S-Function Builder78 : S-Function  Priority=3  Commented=on  FunctionName=GetSpeedReference  SFunctionModules=GetSpeedReference_wrapper  SFunctionDeploymentMode=off  EnableBusSupport=off  mask(S-Function Builder){}
      mask help: Simulink:masks:SFunctionBuilder_MD
      mask init: same as DLL_Demo/S-Function Builder
      settings: CopyFcn=set_param(gcbh,'LinkStatus','none')  OpenFcn=sfunctionwizard(gcbh)
      mask Display:
      | plot(val(:,1),val(:,2))
      | disp(sys)
      | port_label('input',1,'Address')
      | port_label('output',1,'Result')
      | port_label('output',2,'Error')
  S-Function Builder79 : S-Function  Priority=3  Commented=on  FunctionName=GetPowerReference  SFunctionModules=GetPowerReference_wrapper  SFunctionDeploymentMode=off  EnableBusSupport=off  mask(S-Function Builder){}
      mask help: Simulink:masks:SFunctionBuilder_MD
      mask init: same as DLL_Demo/S-Function Builder
      settings: CopyFcn=set_param(gcbh,'LinkStatus','none')  OpenFcn=sfunctionwizard(gcbh)
      mask Display:
      | plot(val(:,1),val(:,2))
      | disp(sys)
      | port_label('input',1,'Address')
      | port_label('output',1,'Result')
      | port_label('output',2,'Error')
  S-Function Builder8 : S-Function  Priority=2  Commented=on  FunctionName=SetSpeedReference  SFunctionModules=SetSpeedReference_wrapper  SFunctionDeploymentMode=off  EnableBusSupport=off  mask(S-Function Builder){}
      mask help: Simulink:masks:SFunctionBuilder_MD
      mask init: same as DLL_Demo/S-Function Builder
      settings: CopyFcn=set_param(gcbh,'LinkStatus','none')  OpenFcn=sfunctionwizard(gcbh)
      mask Display:
      | plot(val(:,1),val(:,2))
      | disp(sys)
      | port_label('input',1,'Address')
      | port_label('input',2,'Value')
      | port_label('output',1,'Result')
      | port_label('output',2,'Error')
  S-Function Builder80 : S-Function  Priority=3  Commented=on  FunctionName=GetPositionReference  SFunctionModules=GetPositionReference_wrapper  SFunctionDeploymentMode=off  EnableBusSupport=off  mask(S-Function Builder){}
      mask help: Simulink:masks:SFunctionBuilder_MD
      mask init: same as DLL_Demo/S-Function Builder
      settings: CopyFcn=set_param(gcbh,'LinkStatus','none')  OpenFcn=sfunctionwizard(gcbh)
      mask Display:
      | plot(val(:,1),val(:,2))
      | disp(sys)
      | port_label('input',1,'Address')
      | port_label('output',1,'Result')
      | port_label('output',2,'Error')
  S-Function Builder81 : S-Function  Priority=3  Commented=on  FunctionName=GetObserverGainBldcPmsm  SFunctionModules=GetObserverGainBldcPmsm_wrapper  SFunctionDeploymentMode=off  EnableBusSupport=off  mask(S-Function Builder){}
      mask help: Simulink:masks:SFunctionBuilder_MD
      mask init: same as DLL_Demo/S-Function Builder
      settings: CopyFcn=set_param(gcbh,'LinkStatus','none')  OpenFcn=sfunctionwizard(gcbh)
      mask Display:
      | plot(val(:,1),val(:,2))
      | disp(sys)
      | port_label('input',1,'Address')
      | port_label('output',1,'Result')
      | port_label('output',2,'Error')
  S-Function Builder82 : S-Function  Priority=3  Commented=on  FunctionName=GetMotorDirection  SFunctionModules=GetMotorDirection_wrapper  SFunctionDeploymentMode=off  EnableBusSupport=off  mask(S-Function Builder){}
      mask help: Simulink:masks:SFunctionBuilder_MD
      mask init: same as DLL_Demo/S-Function Builder
      settings: CopyFcn=set_param(gcbh,'LinkStatus','none')  OpenFcn=sfunctionwizard(gcbh)
      mask Display:
      | plot(val(:,1),val(:,2))
      | disp(sys)
      | port_label('input',1,'Address')
      | port_label('output',1,'Result')
      | port_label('output',2,'Error')
  S-Function Builder83 : S-Function  Priority=3  Commented=on  FunctionName=GetObserverGainBldcPmsmUltrafast  SFunctionModules=GetObserverGainBldcPmsmUltrafast_wrapper  SFunctionDeploymentMode=off  EnableBusSupport=off  mask(S-Function Builder){}
      mask help: Simulink:masks:SFunctionBuilder_MD
      mask init: same as DLL_Demo/S-Function Builder
      settings: CopyFcn=set_param(gcbh,'LinkStatus','none')  OpenFcn=sfunctionwizard(gcbh)
      mask Display:
      | plot(val(:,1),val(:,2))
      | disp(sys)
      | port_label('input',1,'Address')
      | port_label('output',1,'Result')
      | port_label('output',2,'Error')
  S-Function Builder84 : S-Function  Priority=3  Commented=on  FunctionName=GetObserverGainDc  SFunctionModules=GetObserverGainDc_wrapper  SFunctionDeploymentMode=off  EnableBusSupport=off  mask(S-Function Builder){}
      mask help: Simulink:masks:SFunctionBuilder_MD
      mask init: same as DLL_Demo/S-Function Builder
      settings: CopyFcn=set_param(gcbh,'LinkStatus','none')  OpenFcn=sfunctionwizard(gcbh)
      mask Display:
      | plot(val(:,1),val(:,2))
      | disp(sys)
      | port_label('input',1,'Address')
      | port_label('output',1,'Result')
      | port_label('output',2,'Error')
  S-Function Builder85 : S-Function  Priority=3  Commented=on  FunctionName=GetFilterGainBldcPmsm  SFunctionModules=GetFilterGainBldcPmsm_wrapper  SFunctionDeploymentMode=off  EnableBusSupport=off  mask(S-Function Builder){}
      mask help: Simulink:masks:SFunctionBuilder_MD
      mask init: same as DLL_Demo/S-Function Builder
      settings: CopyFcn=set_param(gcbh,'LinkStatus','none')  OpenFcn=sfunctionwizard(gcbh)
      mask Display:
      | plot(val(:,1),val(:,2))
      | disp(sys)
      | port_label('input',1,'Address')
      | port_label('output',1,'Result')
      | port_label('output',2,'Error')
  S-Function Builder86 : S-Function  Priority=3  Commented=on  FunctionName=GetFilterGainBldcPmsmUltrafast  SFunctionModules=GetFilterGainBldcPmsmUltrafast_wrapper  SFunctionDeploymentMode=off  EnableBusSupport=off  mask(S-Function Builder){}
      mask help: Simulink:masks:SFunctionBuilder_MD
      mask init: same as DLL_Demo/S-Function Builder
      settings: CopyFcn=set_param(gcbh,'LinkStatus','none')  OpenFcn=sfunctionwizard(gcbh)
      mask Display:
      | plot(val(:,1),val(:,2))
      | disp(sys)
      | port_label('input',1,'Address')
      | port_label('output',1,'Result')
      | port_label('output',2,'Error')
  S-Function Builder87 : S-Function  Priority=3  Commented=on  FunctionName=Get3PhaseMotorAngle  SFunctionModules=Get3PhaseMotorAngle_wrapper  SFunctionDeploymentMode=off  EnableBusSupport=off  mask(S-Function Builder){}
      mask help: Simulink:masks:SFunctionBuilder_MD
      mask init: same as DLL_Demo/S-Function Builder
      settings: CopyFcn=set_param(gcbh,'LinkStatus','none')  OpenFcn=sfunctionwizard(gcbh)
      mask Display:
      | plot(val(:,1),val(:,2))
      | disp(sys)
      | port_label('input',1,'Address')
      | port_label('output',1,'Result')
      | port_label('output',2,'Error')
  S-Function Builder88 : S-Function  Priority=3  Commented=on  FunctionName=GetEncoderHallCcwOffset  SFunctionModules=GetEncoderHallCcwOffset_wrapper  SFunctionDeploymentMode=off  EnableBusSupport=off  mask(S-Function Builder){}
      mask help: Simulink:masks:SFunctionBuilder_MD
      mask init: same as DLL_Demo/S-Function Builder
      settings: CopyFcn=set_param(gcbh,'LinkStatus','none')  OpenFcn=sfunctionwizard(gcbh)
      mask Display:
      | plot(val(:,1),val(:,2))
      | disp(sys)
      | port_label('input',1,'Address')
      | port_label('output',1,'Result')
      | port_label('output',2,'Error')
  S-Function Builder89 : S-Function  Priority=3  Commented=on  FunctionName=GetEncoderHallCwOffset  SFunctionModules=GetEncoderHallCwOffset_wrapper  SFunctionDeploymentMode=off  EnableBusSupport=off  mask(S-Function Builder){}
      mask help: Simulink:masks:SFunctionBuilder_MD
      mask init: same as DLL_Demo/S-Function Builder
      settings: CopyFcn=set_param(gcbh,'LinkStatus','none')  OpenFcn=sfunctionwizard(gcbh)
      mask Display:
      | plot(val(:,1),val(:,2))
      | disp(sys)
      | port_label('input',1,'Address')
      | port_label('output',1,'Result')
      | port_label('output',2,'Error')
  S-Function Builder9 : S-Function  Priority=2  Commented=on  FunctionName=SetPowerReference  SFunctionModules=SetPowerReference_wrapper  SFunctionDeploymentMode=off  EnableBusSupport=off  mask(S-Function Builder){}
      mask help: Simulink:masks:SFunctionBuilder_MD
      mask init: same as DLL_Demo/S-Function Builder
      settings: CopyFcn=set_param(gcbh,'LinkStatus','none')  OpenFcn=sfunctionwizard(gcbh)
      mask Display: plot(val(:,1),val(:,2)),disp(sys),port_label('input',1,'Address'),port_label('input',2,'Value'),port_label('output',1,'Result'),port_label('output',2,'Error')
  S-Function Builder90 : S-Function  Priority=3  Commented=on  FunctionName=GetUartBaudrate  SFunctionModules=GetUartBaudrate_wrapper  SFunctionDeploymentMode=off  EnableBusSupport=off  mask(S-Function Builder){}
      mask help: Simulink:masks:SFunctionBuilder_MD
      mask init: same as DLL_Demo/S-Function Builder
      settings: CopyFcn=set_param(gcbh,'LinkStatus','none')  OpenFcn=sfunctionwizard(gcbh)
      mask Display:
      | plot(val(:,1),val(:,2))
      | disp(sys)
      | port_label('input',1,'Address')
      | port_label('output',1,'Result')
      | port_label('output',2,'Error')
  S-Function Builder91 : S-Function  Priority=3  Commented=on  FunctionName=GetSpeedAccelerationValue  SFunctionModules=GetSpeedAccelerationValue_wrapper  SFunctionDeploymentMode=off  EnableBusSupport=off  mask(S-Function Builder){}
      mask help: Simulink:masks:SFunctionBuilder_MD
      mask init: same as DLL_Demo/S-Function Builder
      settings: CopyFcn=set_param(gcbh,'LinkStatus','none')  OpenFcn=sfunctionwizard(gcbh)
      mask Display:
      | plot(val(:,1),val(:,2))
      | disp(sys)
      | port_label('input',1,'Address')
      | port_label('output',1,'Result')
      | port_label('output',2,'Error')
  S-Function Builder92 : S-Function  Priority=3  Commented=on  FunctionName=GetSpeedDecelerationValue  SFunctionModules=GetSpeedDecelerationValue_wrapper  SFunctionDeploymentMode=off  EnableBusSupport=off  mask(S-Function Builder){}
      mask help: Simulink:masks:SFunctionBuilder_MD
      mask init: same as DLL_Demo/S-Function Builder
      settings: CopyFcn=set_param(gcbh,'LinkStatus','none')  OpenFcn=sfunctionwizard(gcbh)
      mask Display:
      | plot(val(:,1),val(:,2))
      | disp(sys)
      | port_label('input',1,'Address')
      | port_label('output',1,'Result')
      | port_label('output',2,'Error')
  S-Function Builder93 : S-Function  Priority=3  Commented=on  FunctionName=GetEncoderIndexCounts  SFunctionModules=GetEncoderIndexCounts_wrapper  SFunctionDeploymentMode=off  EnableBusSupport=off  mask(S-Function Builder){}
      mask help: Simulink:masks:SFunctionBuilder_MD
      mask init: same as DLL_Demo/S-Function Builder
      settings: CopyFcn=set_param(gcbh,'LinkStatus','none')  OpenFcn=sfunctionwizard(gcbh)
      mask Display:
      | plot(val(:,1),val(:,2))
      | disp(sys)
      | port_label('input',1,'Address')
      | port_label('output',1,'Result')
      | port_label('output',2,'Error')
  S-Function Builder94 : S-Function  Priority=3  Commented=on  FunctionName=serialIsWorking  SFunctionModules=serialIsWorking_wrapper  SFunctionDeploymentMode=off  EnableBusSupport=off  mask(S-Function Builder){}
      mask help: Simulink:masks:SFunctionBuilder_MD
      mask init: same as DLL_Demo/S-Function Builder
      settings: CopyFcn=set_param(gcbh,'LinkStatus','none')  OpenFcn=sfunctionwizard(gcbh)
      mask Display:
      | plot(val(:,1),val(:,2))
      | disp(sys)
      | port_label('input',1,'Address')
      | port_label('output',1,'Result')
      | port_label('output',2,'Error')
  String Constant : StringConstant  String="\"COM6\""
  String to ASCII : StringToASCII  OutputVectorSize=5
  wires:
  S-Function Builder/1 -> Display1/1
  Constant3/1 -> S-Function Builder/1
  Constant4/1 -> S-Function Builder/2
  S-Function Builder/2 -> Display10/1
  Constant19/1 -> S-Function Builder6/1
  S-Function Builder6/1 -> Display9/1
  S-Function Builder6/2 -> Display11/1
  Constant18/1 -> S-Function Builder5/1
  String to ASCII/1 -> S-Function Builder5/2
  Constant12/1 -> S-Function Builder5/4
  Constant13/1 -> S-Function Builder5/5
  S-Function Builder5/1 -> Display5/1
  Constant1/1 -> S-Function Builder5/3
  String Constant/1 -> String to ASCII/1
  S-Function Builder1/1 -> Display2/1
  Constant2/1 -> S-Function Builder1/1
  S-Function Builder1/2 -> Display3/1
  Constant5/1 -> S-Function Builder1/2
  S-Function Builder2/2 -> Display6/1
  S-Function Builder2/1 -> Display4/1
  Constant7/1 -> S-Function Builder2/2
  Constant6/1 -> S-Function Builder2/1
  Constant8/1 -> S-Function Builder3/1
  S-Function Builder3/2 -> Display7/1
  S-Function Builder3/1 -> Display8/1
  S-Function Builder4/1 -> Display12/1
  Constant10/1 -> S-Function Builder4/2
  S-Function Builder4/2 -> Display13/1
  Constant9/1 -> S-Function Builder4/1
  S-Function Builder7/1 -> Display15/1
  S-Function Builder7/2 -> Display14/1
  Constant11/1 -> S-Function Builder7/1
  Constant15/1 -> S-Function Builder8/1
  Constant14/1 -> S-Function Builder8/2
  S-Function Builder8/1 -> Display16/1
  S-Function Builder8/2 -> Display17/1
  S-Function Builder9/2 -> Display19/1
  Constant16/1 -> S-Function Builder9/2
  Constant17/1 -> S-Function Builder9/1
  S-Function Builder9/1 -> Display18/1
  S-Function Builder10/1 -> Display20/1
  Constant21/1 -> S-Function Builder10/1
  Constant20/1 -> S-Function Builder10/2
  S-Function Builder10/2 -> Display21/1
  S-Function Builder11/2 -> Display23/1
  Constant23/1 -> S-Function Builder11/1
  S-Function Builder11/1 -> Display22/1
  S-Function Builder12/2 -> Display25/1
  Constant22/1 -> S-Function Builder12/2
  Constant24/1 -> S-Function Builder12/1
  S-Function Builder12/1 -> Display24/1
  S-Function Builder13/1 -> Display26/1
  Constant26/1 -> S-Function Builder13/1
  Constant25/1 -> S-Function Builder13/2
  S-Function Builder13/2 -> Display27/1
  Constant28/1 -> S-Function Builder14/1
  S-Function Builder14/1 -> Display28/1
  S-Function Builder14/2 -> Display29/1
  Constant27/1 -> S-Function Builder14/2
  Constant29/1 -> S-Function Builder15/2
  S-Function Builder15/2 -> Display31/1
  S-Function Builder15/1 -> Display30/1
  Constant30/1 -> S-Function Builder15/1
  Constant32/1 -> S-Function Builder16/1
  S-Function Builder16/1 -> Display32/1
  S-Function Builder16/2 -> Display33/1
  Constant31/1 -> S-Function Builder16/2
  Constant33/1 -> S-Function Builder17/2
  S-Function Builder17/1 -> Display34/1
  Constant34/1 -> S-Function Builder17/1
  S-Function Builder17/2 -> Display35/1
  S-Function Builder18/2 -> Display37/1
  Constant35/1 -> S-Function Builder18/2
  Constant36/1 -> S-Function Builder18/1
  S-Function Builder18/1 -> Display36/1
  S-Function Builder19/1 -> Display38/1
  Constant38/1 -> S-Function Builder19/1
  S-Function Builder19/2 -> Display39/1
  Constant37/1 -> S-Function Builder19/2
  Constant40/1 -> S-Function Builder20/1
  S-Function Builder20/1 -> Display40/1
  S-Function Builder20/2 -> Display41/1
  Constant39/1 -> S-Function Builder20/2
  S-Function Builder21/2 -> Display43/1
  Constant41/1 -> S-Function Builder21/2
  S-Function Builder21/1 -> Display42/1
  Constant42/1 -> S-Function Builder21/1
  Constant43/1 -> S-Function Builder22/1
  S-Function Builder22/2 -> Display45/1
  S-Function Builder22/1 -> Display44/1
  Constant44/1 -> S-Function Builder23/2
  S-Function Builder23/1 -> Display46/1
  S-Function Builder23/2 -> Display47/1
  Constant45/1 -> S-Function Builder23/1
  S-Function Builder24/2 -> Display49/1
  Constant46/1 -> S-Function Builder24/1
  S-Function Builder24/1 -> Display48/1
  Constant48/1 -> S-Function Builder25/1
  S-Function Builder25/1 -> Display50/1
  S-Function Builder25/2 -> Display51/1
  Constant47/1 -> S-Function Builder25/2
  Constant50/1 -> S-Function Builder26/1
  S-Function Builder26/1 -> Display52/1
  S-Function Builder26/2 -> Display53/1
  Constant49/1 -> S-Function Builder26/2
  S-Function Builder27/1 -> Display54/1
  Constant51/1 -> S-Function Builder27/2
  Constant52/1 -> S-Function Builder27/1
  S-Function Builder27/2 -> Display55/1
  S-Function Builder28/1 -> Display56/1
  S-Function Builder28/2 -> Display57/1
  Constant54/1 -> S-Function Builder28/1
  Constant53/1 -> S-Function Builder28/2
  S-Function Builder29/1 -> Display58/1
  S-Function Builder29/2 -> Display59/1
  Constant56/1 -> S-Function Builder29/1
  Constant55/1 -> S-Function Builder29/2
  S-Function Builder30/2 -> Display61/1
  S-Function Builder30/1 -> Display60/1
  Constant57/1 -> S-Function Builder30/2
  Constant58/1 -> S-Function Builder30/1
  S-Function Builder31/2 -> Display63/1
  S-Function Builder31/1 -> Display62/1
  Constant59/1 -> S-Function Builder31/2
  Constant60/1 -> S-Function Builder31/1
  Constant61/1 -> S-Function Builder32/2
  S-Function Builder32/2 -> Display65/1
  Constant62/1 -> S-Function Builder32/1
  S-Function Builder32/1 -> Display64/1
  S-Function Builder33/1 -> Display66/1
  S-Function Builder33/2 -> Display67/1
  Constant63/1 -> S-Function Builder33/1
  Constant64/1 -> S-Function Builder34/1
  S-Function Builder34/1 -> Display68/1
  S-Function Builder34/2 -> Display69/1
  S-Function Builder35/1 -> Display70/1
  Constant66/1 -> S-Function Builder35/1
  Constant65/1 -> S-Function Builder35/2
  S-Function Builder35/2 -> Display71/1
  Constant67/1 -> S-Function Builder36/2
  Constant68/1 -> S-Function Builder36/1
  S-Function Builder36/2 -> Display73/1
  S-Function Builder36/1 -> Display72/1
  Constant69/1 -> S-Function Builder37/2
  S-Function Builder37/2 -> Display75/1
  S-Function Builder37/1 -> Display74/1
  Constant70/1 -> S-Function Builder37/1
  Constant72/1 -> S-Function Builder38/1
  S-Function Builder38/2 -> Display77/1
  Constant71/1 -> S-Function Builder38/2
  S-Function Builder38/1 -> Display76/1
  Constant74/1 -> S-Function Builder39/1
  Constant73/1 -> S-Function Builder39/2
  S-Function Builder39/2 -> Display79/1
  S-Function Builder39/1 -> Display78/1
  S-Function Builder40/1 -> Display80/1
  Constant75/1 -> S-Function Builder40/2
  Constant76/1 -> S-Function Builder40/1
  S-Function Builder40/2 -> Display81/1
  S-Function Builder41/2 -> Display83/1
  Constant77/1 -> S-Function Builder41/2
  Constant78/1 -> S-Function Builder41/1
  S-Function Builder41/1 -> Display82/1
  S-Function Builder42/1 -> Display84/1
  Constant79/1 -> S-Function Builder42/2
  Constant80/1 -> S-Function Builder42/1
  S-Function Builder42/2 -> Display85/1
  S-Function Builder43/2 -> Display87/1
  Constant82/1 -> S-Function Builder43/1
  S-Function Builder43/1 -> Display86/1
  Constant81/1 -> S-Function Builder43/2
  Constant84/1 -> S-Function Builder44/1
  S-Function Builder44/1 -> Display88/1
  Constant83/1 -> S-Function Builder44/2
  S-Function Builder44/2 -> Display89/1
  S-Function Builder45/2 -> Display91/1
  Constant86/1 -> S-Function Builder45/1
  Constant85/1 -> S-Function Builder45/2
  S-Function Builder45/1 -> Display90/1
  Constant87/1 -> S-Function Builder46/2
  Constant88/1 -> S-Function Builder46/1
  S-Function Builder46/1 -> Display92/1
  S-Function Builder46/2 -> Display93/1
  Constant89/1 -> S-Function Builder47/1
  S-Function Builder47/2 -> Display94/1
  S-Function Builder47/1 -> Display95/1
  S-Function Builder48/1 -> Display97/1
  S-Function Builder48/2 -> Display96/1
  Constant90/1 -> S-Function Builder48/1
  Constant91/1 -> S-Function Builder49/1
  S-Function Builder49/2 -> Display98/1
  S-Function Builder49/1 -> Display99/1
  S-Function Builder50/2 -> Display100/1
  S-Function Builder50/1 -> Display101/1
  Constant92/1 -> S-Function Builder50/1
  Constant93/1 -> S-Function Builder51/1
  S-Function Builder51/2 -> Display102/1
  S-Function Builder51/1 -> Display103/1
  S-Function Builder52/2 -> Display104/1
  Constant94/1 -> S-Function Builder52/1
  S-Function Builder52/1 -> Display105/1
  S-Function Builder53/1 -> Display107/1
  S-Function Builder53/2 -> Display106/1
  Constant95/1 -> S-Function Builder53/1
  Constant96/1 -> S-Function Builder54/1
  S-Function Builder54/2 -> Display108/1
  S-Function Builder54/1 -> Display109/1
  Constant97/1 -> S-Function Builder55/1
  S-Function Builder55/2 -> Display110/1
  S-Function Builder55/1 -> Display111/1
  Constant98/1 -> S-Function Builder56/1
  S-Function Builder56/2 -> Display112/1
  S-Function Builder56/1 -> Display113/1
  Constant99/1 -> S-Function Builder57/1
  S-Function Builder57/2 -> Display114/1
  S-Function Builder57/1 -> Display115/1
  S-Function Builder58/2 -> Display116/1
  S-Function Builder58/1 -> Display117/1
  Constant100/1 -> S-Function Builder58/1
  Constant101/1 -> S-Function Builder59/1
  S-Function Builder59/1 -> Display119/1
  S-Function Builder59/2 -> Display118/1
  S-Function Builder60/2 -> Display120/1
  S-Function Builder60/1 -> Display121/1
  Constant102/1 -> S-Function Builder60/1
  Constant103/1 -> S-Function Builder61/1
  S-Function Builder61/2 -> Display122/1
  S-Function Builder61/1 -> Display123/1
  S-Function Builder62/1 -> Display125/1
  S-Function Builder62/2 -> Display124/1
  Constant104/1 -> S-Function Builder62/1
  S-Function Builder63/1 -> Display127/1
  S-Function Builder63/2 -> Display126/1
  Constant105/1 -> S-Function Builder63/1
  S-Function Builder64/1 -> Display129/1
  S-Function Builder64/2 -> Display128/1
  Constant106/1 -> S-Function Builder64/1
  S-Function Builder65/2 -> Display130/1
  Constant107/1 -> S-Function Builder65/1
  S-Function Builder66/1 -> Display133/1
  S-Function Builder66/2 -> Display132/1
  Constant108/1 -> S-Function Builder66/1
  Constant109/1 -> S-Function Builder67/1
  S-Function Builder67/2 -> Display134/1
  S-Function Builder67/1 -> Display135/1
  Constant110/1 -> S-Function Builder68/1
  S-Function Builder68/2 -> Display136/1
  S-Function Builder68/1 -> Display137/1
  Constant111/1 -> S-Function Builder69/1
  S-Function Builder69/2 -> Display138/1
  S-Function Builder69/1 -> Display139/1
  Constant112/1 -> S-Function Builder70/1
  S-Function Builder70/2 -> Display140/1
  S-Function Builder70/1 -> Display141/1
  S-Function Builder71/1 -> Display143/1
  Constant113/1 -> S-Function Builder71/1
  S-Function Builder71/2 -> Display142/1
  S-Function Builder72/1 -> Display145/1
  Constant114/1 -> S-Function Builder72/1
  S-Function Builder72/2 -> Display144/1
  S-Function Builder73/1 -> Display147/1
  S-Function Builder73/2 -> Display146/1
  Constant115/1 -> S-Function Builder73/1
  S-Function Builder74/1 -> Display149/1
  S-Function Builder74/2 -> Display148/1
  Constant116/1 -> S-Function Builder74/1
  S-Function Builder75/1 -> Display151/1
  S-Function Builder75/2 -> Display150/1
  Constant117/1 -> S-Function Builder75/1
  S-Function Builder76/1 -> Display153/1
  S-Function Builder76/2 -> Display152/1
  Constant118/1 -> S-Function Builder76/1
  S-Function Builder77/2 -> Display154/1
  Constant119/1 -> S-Function Builder77/1
  S-Function Builder77/1 -> Display155/1
  S-Function Builder78/1 -> Display157/1
  Constant120/1 -> S-Function Builder78/1
  S-Function Builder78/2 -> Display156/1
  S-Function Builder79/2 -> Display158/1
  Constant121/1 -> S-Function Builder79/1
  S-Function Builder80/1 -> Display161/1
  S-Function Builder80/2 -> Display160/1
  S-Function Builder79/1 -> Display159/1
  Constant122/1 -> S-Function Builder80/1
  Constant124/1 -> S-Function Builder82/1
  S-Function Builder82/1 -> Display165/1
  S-Function Builder82/2 -> Display164/1
  S-Function Builder81/1 -> Display163/1
  Constant123/1 -> S-Function Builder81/1
  S-Function Builder81/2 -> Display162/1
  Constant125/1 -> S-Function Builder83/1
  S-Function Builder83/2 -> Display166/1
  S-Function Builder83/1 -> Display167/1
  Constant126/1 -> S-Function Builder84/1
  S-Function Builder84/2 -> Display168/1
  S-Function Builder84/1 -> Display169/1
  Constant127/1 -> S-Function Builder85/1
  S-Function Builder85/2 -> Display170/1
  S-Function Builder85/1 -> Display171/1
  Constant128/1 -> S-Function Builder86/1
  S-Function Builder86/2 -> Display172/1
  S-Function Builder86/1 -> Display173/1
  Constant129/1 -> S-Function Builder87/1
  S-Function Builder87/2 -> Display174/1
  S-Function Builder87/1 -> Display175/1
  Constant130/1 -> S-Function Builder88/1
  S-Function Builder88/2 -> Display176/1
  S-Function Builder88/1 -> Display177/1
  Constant131/1 -> S-Function Builder89/1
  S-Function Builder89/2 -> Display178/1
  S-Function Builder89/1 -> Display179/1
  Constant132/1 -> S-Function Builder90/1
  S-Function Builder90/2 -> Display180/1
  S-Function Builder90/1 -> Display181/1
  S-Function Builder91/1 -> Display183/1
  Constant133/1 -> S-Function Builder91/1
  S-Function Builder91/2 -> Display182/1
  S-Function Builder92/1 -> Display185/1
  Constant134/1 -> S-Function Builder92/1
  S-Function Builder92/2 -> Display184/1
  Constant135/1 -> S-Function Builder93/1
  S-Function Builder93/1 -> Display187/1
  S-Function Builder93/2 -> Display186/1
  S-Function Builder94/2 -> Display188/1
  S-Function Builder94/1 -> Display189/1
  Constant136/1 -> S-Function Builder94/1
  S-Function Builder65/1 -> Display131/1
